simulink model "dragFallBall"  (R2018a)
settings: Solver=ode45  StartTime=0.0  StopTime=10.0  RelTol=1e-3  EnableMultiTasking=on
PreLoadFcn:
  | Cdrag = 1;
  | m = 1;
settings Model: Creator=jrivitus  LastModifiedBy=bneiswan
settings DataIOCC: LimitDataPoints=on  SaveFormat=Array
settings OptimizationCC: ExpressionDepthLimit=2147483647  InitFltsAndDblsToZero=on  LifeSpan=inf
settings DebuggingCC: UnderspecifiedInitializationDetection=Classic  MergeDetectMultiDrivingBlocksExec=none  ParameterPrecisionLossMsg=none  FcnCallInpInsideContextMsg=warning  AllowSymbolicDim=off  StateNameClashWarn=warning  SFUnexpectedBacktrackingDiag=warning  SFNoUnconditionalDefaultTransitionDiag=warning  SFExecutionAtInitializationDiag=none
settings HardwareCC: ProdBitPerPointer=32  ProdBitPerSizeT=32  ProdBitPerPtrDiffT=32  ProdLargestAtomicFloat=None  ProdIntDivRoundTo=Undefined  ProdEndianess=Unspecified  ProdWordSize=32  ProdHWDeviceType=32-bit Generic
settings ModelReferenceCC: PropagateSignalLabelsOutOfModel=off
settings CodeAppCC: StateflowObjectComments=on
settings GRTTargetCC: TargetLangStandard=C89/C90 (ANSI)  GeneratePreprocessorConditionals=Disable all  CombineOutputUpdateFcns=off  GRTInterface=on
settings ConfigComp: CovMetricSettings=dw  CovHtmlReporting=on  CovSaveCumulativeToWorkspaceVar=on  CovSaveSingleToWorkspaceVar=on  CovExternalEMLEnable=off  CovSFcnEnable=off

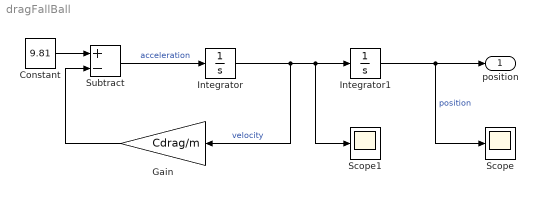
== system dragFallBall ==
  Constant : Constant  Value=9.81
  Gain : Gain  Gain=Cdrag/m
  Integrator : Integrator  InitialCondition=-50
      settings: AttributesFormatString=v0 = %<InitialCondition>
  Integrator1 : Integrator
      settings: AttributesFormatString=x0 = %<InitialCondition>
  Scope : Scope
  Scope1 : Scope
  Subtract : Sum  Inputs=+-
  position : Outport
  wires:
  Subtract/1 -> Integrator/1  "acceleration"
  Integrator/1 -> Gain/1, Integrator1/1, Scope1/1  "velocity"
  Integrator1/1 -> position/1, Scope/1  "position"
  Constant/1 -> Subtract/1
  Gain/1 -> Subtract/2
